simulink model "B1D"  (R2019a)
settings: Solver=ode1  StartTime=0.0  StopTime=60  FixedStep=0.00001  RelTol=1e-3  AbsTol=1e-3
settings Model: Creator=Mehmet Şahin  LastModifiedBy=Mehmet Şahin
settings SolverCC: AutoScaleAbsTol=off
settings DataIOCC: LimitDataPoints=on  MaxDataPoints=10000
settings OptimizationCC: LifeSpan=inf
settings DebuggingCC: AllowSymbolicDim=off  PregeneratedLibrarySubsystemCodeDiagnostic=none  SFUnexpectedBacktrackingDiag=warning  SFNoUnconditionalDefaultTransitionDiag=warning  SFExecutionAtInitializationDiag=none  ArithmeticOperatorsInVariantConditions=warning
settings SFSimCC: SimUseLocalCustomCode=off
settings RTWCC: RTWUseLocalCustomCode=off
settings CodeAppCC: StateflowObjectComments=on
settings GRTTargetCC: TargetLangStandard=C89/C90 (ANSI)  GeneratePreprocessorConditionals=Disable all
settings ConfigComp: CovMetricSettings=dw  CovHtmlReporting=on  CovSaveCumulativeToWorkspaceVar=on  CovSaveSingleToWorkspaceVar=on  CovExternalEMLEnable=off  CovSFcnEnable=off
settings SimscapeCC: SimscapeLogType=all  SimscapeLogDataHistory=10000

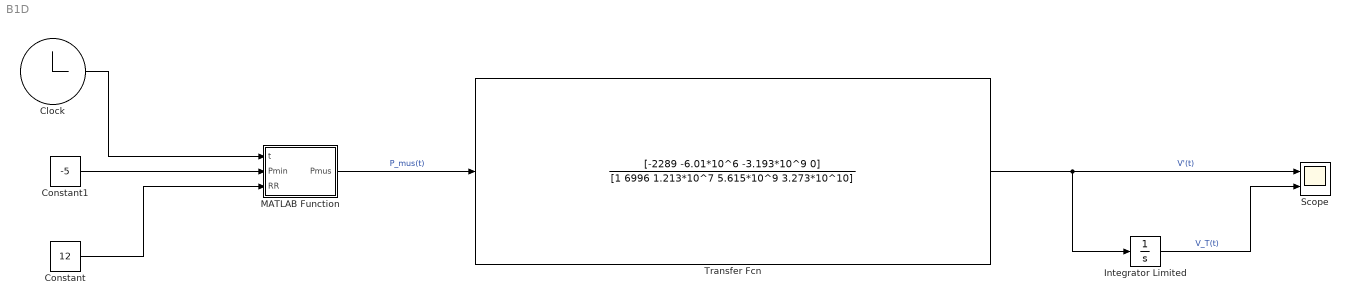
== system B1D ==
  Clock : Clock
      settings: Decimation=5
  Constant : Constant  Value=12
  Constant1 : Constant  Value=-5
  Integrator Limited : Integrator  LimitOutput=on  UpperSaturationLimit=1  LowerSaturationLimit=0
  MATLAB Function : MATLAB Function  TreatAsAtomicUnit=on
  Scope : Scope  NumInputPorts=2
  Transfer Fcn : TransferFcn  Numerator=[-2289 -6.01*10^6 -3.193*10^9 0]  Denominator=[1 6996 1.213*10^7 5.615*10^9 3.273*10^10]
  wires:
  MATLAB Function/1(Pmus) -> Transfer Fcn/1  "P_mus(t)"
  Clock/1 -> MATLAB Function/1(t)
  Constant/1 -> MATLAB Function/3(RR)
  Constant1/1 -> MATLAB Function/2(Pmin)
  Transfer Fcn/1 -> Integrator Limited/1, Scope/1  "V'(t)"
  Integrator Limited/1 -> Scope/2  "V_T(t)"

== matlab function B1D/MATLAB Function ==
  data: t input; Pmin input; RR input; Pmus output
function Pmus = fcn(t, Pmin, RR)
IEratio = 1/2;
T=(60/RR);
Te = T / (IEratio + 1);
Ti = IEratio * Te;
tau=Te/10;
if (rem(t,T)) < Ti
u=Pmin*(T*rem(t,T)-rem(t,T)^2)/(Ti*Te);
else
u=Pmin*(exp(-(rem(t,T)-Ti)/tau)-exp(-Te/tau))/(1-exp(-Te/tau));
end
Pmus = u;
end
